simulink model "Lab1_parameter_estimation_student"  (R2025b)
settings: Solver=FixedStepAuto  StartTime=0.0  StopTime=inf  FixedStep=0.001  RelTol=1e-3
values from neighbouring files (symbols this model uses):
  motor_B = 0.000160622    [Lab1_motor_params_student.m]
  motor_Eff = 0.99657    [Lab1_motor_params_student.m]
  motor_J = 0.000086355    (= 8.6355e-05)    [Lab1_motor_params_student.m]
  motor_Ke = 0.030185667    [Lab1_motor_params_student.m]
  motor_L = 0.2304    [Lab1_motor_params_student.m]
  motor_R = 2.418    [Lab1_motor_params_student.m]
libraries: simulink x4
settings Model: Creator=tanawatp  LastModifiedBy=User
settings DataIOCC: OutputOption=AdditionalOutputTimes  OutputTimes=SDO_OutputTimes  ReturnWorkspaceOutputsName=SDOSimTest_Log
settings RTWCC: GPUComputeCapability=3.5

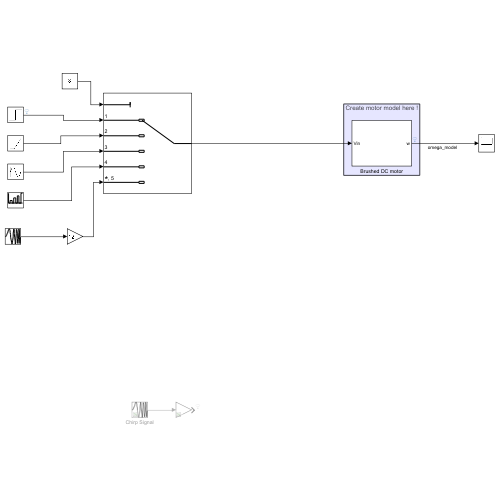
[thumbnail: Simulink's stored preview of the top-level diagram]
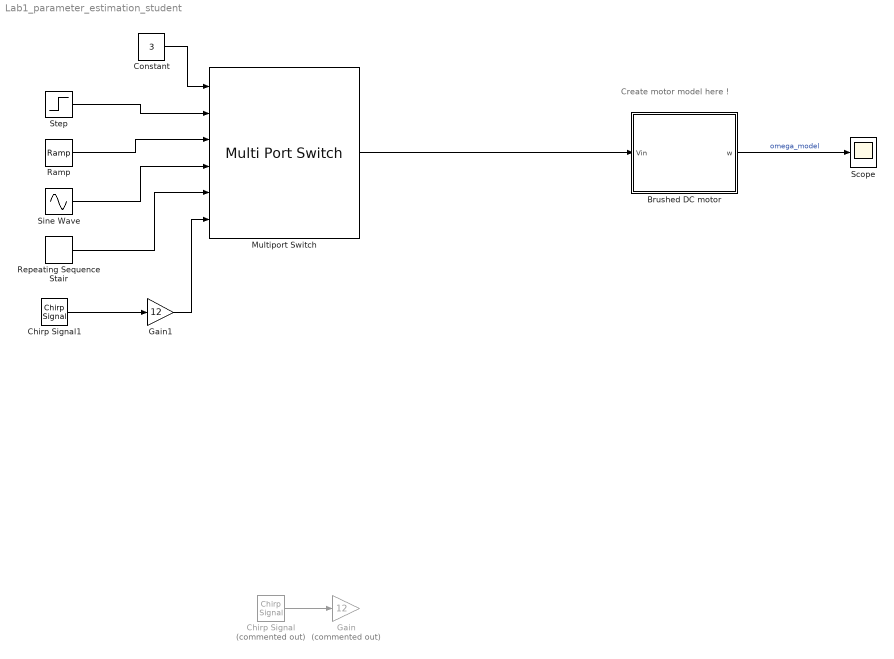
== system Lab1_parameter_estimation_student ==
  note: Create motor model here !
  Brushed DC motor : Subsystem
  Chirp Signal : simulink/Sources/Chirp Signal  Commented=on  f1=0.1  T=40  f2=5
  Chirp Signal1 : simulink/Sources/Chirp Signal  f1=0.1  T=30  f2=1
  Constant : Constant  Value=3
  Gain : Gain  Commented=on  Gain=12
  Gain1 : Gain  Gain=12
  Multiport Switch : MultiPortSwitch  Inputs=5  SaturateOnIntegerOverflow=off  InputSameDT=off
  Ramp : simulink/Sources/Ramp  slope=0.48  start=0  InitialOutput=0
  Repeating Sequence Stair : simulink/Sources/Repeating Sequence Stair  OutValues=[0 3 0 6 0 9 0 12].'  tsamp=2.778  OutMin=[]  OutMax=[]  OutDataTypeStr=double  OutputDataTypeScalingMode=double  OutDataType=fixdt(0,8)  ConRadixGroup=Best Precision: Vector-wise  OutScaling=2^-12
  Scope : Scope
      settings: ActiveDisplayYMinimum=-26.38033  ActiveDisplayYMaximum=237.42293
  Sine Wave : Sin  Amplitude=12  Frequency=pi  SampleTime=0
  Step : Step  After=12  SampleTime=0
  wires:
  Brushed DC motor/1(w) -> Scope/1  "omega_model"
  Chirp Signal/1 -> Gain/1
  Repeating Sequence Stair/1 -> Multiport Switch/5
  Multiport Switch/1 -> Brushed DC motor/1(Vin)
  Ramp/1 -> Multiport Switch/3
  Step/1 -> Multiport Switch/2
  Chirp Signal1/1 -> Gain1/1
  Constant/1 -> Multiport Switch/1
  Gain1/1 -> Multiport Switch/6
  Sine Wave/1 -> Multiport Switch/4

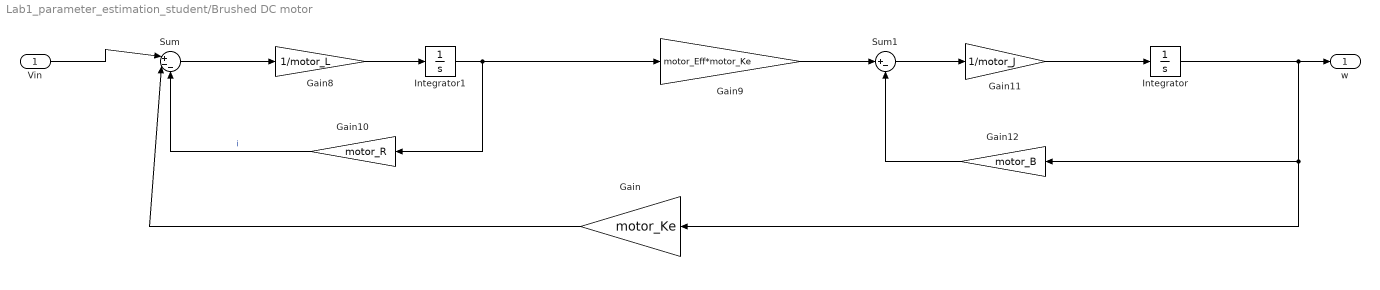
== system Lab1_parameter_estimation_student/Brushed DC motor ==
  Vin : Inport
  Gain : Gain  Gain=motor_Ke
  Gain10 : Gain  Gain=motor_R
  Gain11 : Gain  Gain=1/motor_J
  Gain12 : Gain  Gain=motor_B
  Gain8 : Gain  Gain=1/motor_L
  Gain9 : Gain  Gain=motor_Eff*motor_Ke
  Integrator : Integrator
  Integrator1 : Integrator
  Sum : Sum  Inputs=|+--
  Sum1 : Sum  Inputs=|+-
  w : Outport
  wires:
  Vin/1 -> Sum/1
  Sum/1 -> Gain8/1
  Gain8/1 -> Integrator1/1
  Integrator1/1 -> Gain9/1, Gain10/1
  Gain11/1 -> Integrator/1
  Integrator/1 -> Gain12/1, Gain/1, w/1
  Gain/1 -> Sum/2
  Gain10/1 -> Sum/3  "i"
  Gain9/1 -> Sum1/1
  Sum1/1 -> Gain11/1
  Gain12/1 -> Sum1/2
